simulink model "QP_lev2"  (R2022b)
settings: Solver=ode1  StartTime=0.0  StopTime=T_run  FixedStep=Ts  MaxStep=0.001  MinStep=0.001  RelTol=1e-3
InitFcn:
  | IMPC_Controller_simulink_initial
StopFcn:
  | Analyze
values from neighbouring files (symbols this model uses):
  A = [    A1       A2 ... (first row only)    [IMPC_Controller_simulink_initial.m]
  A_QP = reshape([W1;W2;W3;W4;I_bar]',m*n,1)    [IMPC_Controller_simulink_initial.m]
  B = [        B1 ... (first row only)    [IMPC_Controller_simulink_initial.m]
  D_bar_inv = inv(D_bar)    [IMPC_Controller_simulink_initial.m]
  d_gl = 1.0000    (= 1)    [IMPC_Controller_simulink_initial.m]
  d_l = 1.0000    (= 1)    [IMPC_Controller_simulink_initial.m]
  d_m_plus_d_g = 2.2036    [IMPC_Controller_simulink_initial.m]
  H_QP = reshape(H,((Nc))^2,1)    [IMPC_Controller_simulink_initial.m]
  K_b = Kb_coe*362    (= 362)    [IMPC_Controller_simulink_initial.m]
  L1_tilde = L1_bar*A_tilde    [IMPC_Controller_simulink_initial.m]
  L2_tilde = L2_bar*A_tilde    [IMPC_Controller_simulink_initial.m]
  L3_tilde = L3_bar*A_tilde    [IMPC_Controller_simulink_initial.m]
  L4_tilde = L4_bar*A_tilde    [IMPC_Controller_simulink_initial.m]
  lb_QP = dtau_min_bar    [IMPC_Controller_simulink_initial.m]
  lbA_QP_ini = [ repmat(q_min,N+1,1) ... (first row only)    [IMPC_Controller_simulink_initial.m]
  M_bar_inv = inv(M_bar)    [IMPC_Controller_simulink_initial.m]
  N = 10    [IMPC_Controller_simulink_initial.m]
  Q_const_pos_error = 8000    [IMPC_Controller_simulink_initial.m]
  Q_const_theta_error = 0    [IMPC_Controller_simulink_initial.m]
  Q_const_vel_error = 50    [IMPC_Controller_simulink_initial.m]
  q_sim_ini = q_ini    [IMPC_Controller_simulink_initial.m]
  R_const = 0.01    [IMPC_Controller_simulink_initial.m]
  tau_sim_ini = 0    [IMPC_Controller_simulink_initial.m]
  Ts = 0.001    [IMPC_Controller_simulink_initial.m]
  ub_QP = dtau_max_bar    [IMPC_Controller_simulink_initial.m]
  ubA_QP_ini = [ repmat(q_max,N+1,1) ... (first row only)    [IMPC_Controller_simulink_initial.m]
  var_u = 0    [IMPC_Controller_simulink_initial.m]
  var_y = 1e-12    [IMPC_Controller_simulink_initial.m]
  X_bar_sim_ini = [q_bar_sim_ini;theta_sim_ini;theta_d_sim_ini]    [IMPC_Controller_simulink_initial.m]
undefined symbols (not defined in the file or in its folder): C, D, exJoint, Xr
libraries: simulink x9, cstblocks x4
settings Model: PauseTimes=7.5  Creator=ywang  LastModifiedBy=zheng
settings SolverCC: InitialStep=0.001  AlgebraicLoopSolver=LineSearch
settings DataIOCC: ReturnWorkspaceOutputs=off
settings DebuggingCC: UnconnectedInputMsg=warning  UnconnectedOutputMsg=warning  UnconnectedLineMsg=warning  PregeneratedLibrarySubsystemCodeDiagnostic=none  SFMachineParentedDataDiag=warning  ArithmeticOperatorsInVariantConditions=warning
settings ModelReferenceCC: EnableRefExpFcnMdlSchedulingChecks=on
settings SFSimCC: SimUseLocalCustomCode=off  CustomCodeUndefinedFunction=UseInterfaceOnly
settings RTWCC: RTWUseLocalCustomCode=off  DLArmComputeVersion=19.05
settings CodeAppCC: StateflowObjectComments=on

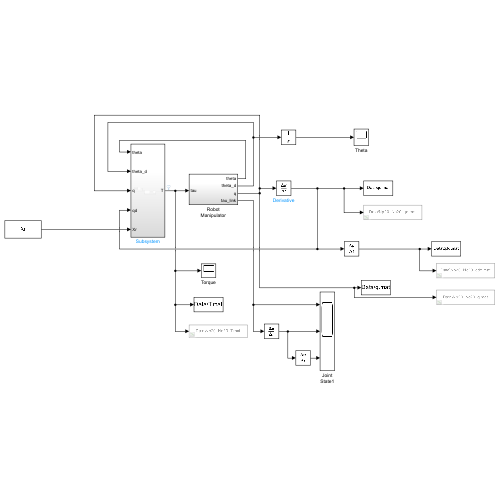
[thumbnail: Simulink's stored preview of the top-level diagram]
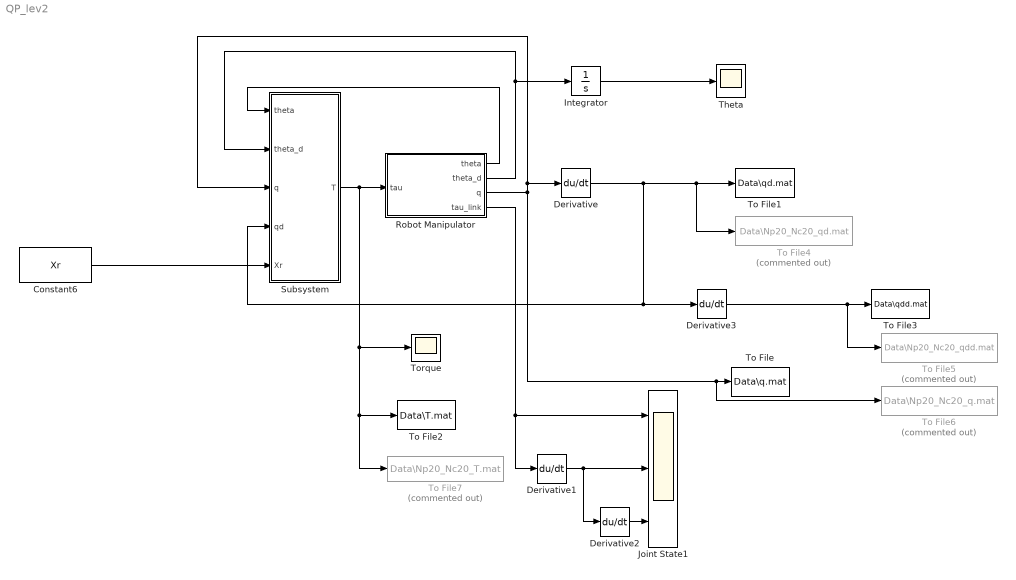
== system QP_lev2 ==
  Constant6 : Constant  Value=Xr
  Derivative{,1..3} (4 alike) : Derivative
  Integrator : Integrator
  Joint State1 : Scope  NumInputPorts=3
  Robot Manipulator : Subsystem
  Subsystem : Subsystem
  Theta : Scope
  To File : ToFile  Filename=Data\q.mat  MatrixName=q
  To File1 : ToFile  Filename=Data\qd.mat  MatrixName=qd
  To File2 : ToFile  Filename=Data\T.mat  MatrixName=T
  To File3 : ToFile  Filename=Data\qdd.mat  MatrixName=qdd
  To File4 : ToFile  Commented=on  Filename=Data\Np20_Nc20_qd.mat  MatrixName=Np20_Nc20_qd
  To File5 : ToFile  Commented=on  Filename=Data\Np20_Nc20_qdd.mat  MatrixName=Np20_Nc20_qdd
  To File6 : ToFile  Commented=on  Filename=Data\Np20_Nc20_q.mat  MatrixName=Np20_Nc20_q
  To File7 : ToFile  Commented=on  Filename=Data\Np20_Nc20_T.mat  MatrixName=Np20_Nc20_T
  Torque : Scope
  wires:
  Subsystem/1(T) -> To File7/1, To File2/1, Torque/1, Robot Manipulator/1(tau)
  Derivative/1 -> Derivative3/1, Subsystem/4(qd), To File4/1, To File1/1
  Robot Manipulator/3(q) -> Subsystem/3(q), Derivative/1, To File/1, To File6/1
  Constant6/1 -> Subsystem/5(Xr)
  Robot Manipulator/2(theta_d) -> Subsystem/2(theta_d), Integrator/1
  Integrator/1 -> Theta/1
  Robot Manipulator/4(tau_link) -> Derivative1/1, Joint State1/1
  Derivative1/1 -> Joint State1/2, Derivative2/1
  Derivative2/1 -> Joint State1/3
  Derivative3/1 -> To File5/1, To File3/1
  Robot Manipulator/1(theta) -> Subsystem/1(theta)

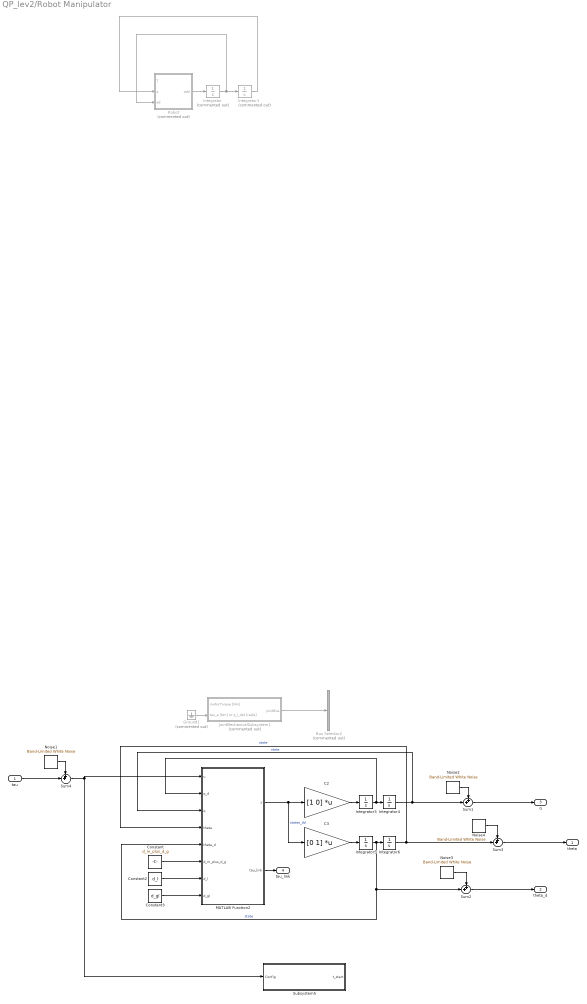
== system QP_lev2/Robot Manipulator ==
  tau : Inport  PortDimensions=1
  Bus Selector2 : BusSelector  Commented=on  OutputSignals=LinkPos,MotorPos,Torque
  C2 : Gain  Gain=[1 0]  Multiplication=Matrix(K*u)
  C3 : Gain  Gain=[0 1]  Multiplication=Matrix(K*u)
  Constant : Constant  Value=d_m_plus_d_g
  Constant2 : Constant  Value=d_l
  Constant3 : Constant  Value=d_gl
  Ground1 : Ground  Commented=on
  Integrator : Integrator  Commented=on  InitialCondition=[0;0;0]  ContinuousStateAttributes='velocity'
  Integrator1 : Integrator  Commented=on  InitialCondition=q_sim_ini  ContinuousStateAttributes='position'
  Integrator{3..6} (4 alike) : Integrator
  JointMechanicalSubsystem1 : Subsystem  Commented=on  AncestorBlock=cjt_library_models/Joint models/JointMechanicalSubsystem  mask(jointMechanicalSubsystem){jointObj=exJoint, fc_vel=1000, fc_torque=1000, input_delay=0, output_delay=1, quantize=off, quantize_bits=19, input_noise_enabled=off, output_noise_enabled=off, var_u=0, var_y=1.8e-10}
      mask prompts: jointObj "Joint Object"; fc_vel "Velocity filter cut-off frequency [Hz]"; fc_torque "Torque filter cut-off frequency [Hz]"; input_delay "Motor torque input delay (num samples of Ts)"; output_delay "Output delay (num samples of Ts)"; quantize "Quantize measurements"; quantize_bits "Quantization bits"; input_noise_enabled "Enable input noise"; output_noise_enabled "Enable measurement noise"; var_u "Input noise variance"; var_y "Measurement noise variance"
      mask help:
      | This block implements the mechanical dynamics of the actuator.
      |
      | For more information, see the > Help <.
      mask init:
      | % Get linear dynamics matrices
      | [A, B, C, D, I, R, K] = jointObj.getDynamicsMatrices();
      | 
      | % Build B matrix for nonlinear components
      | B_nonlinear = [zeros([size(B,1)-size(I,1),1]); 1./diag(I)];
      | 
      | % Get other properties
      | Ts      = jointObj.Ts;
      | Ts_elec = jointObj.Ts_elec;
      | k_b     = jointObj.k_b;
      | k_t     = jointObj.k_t;
      | n       = jointObj.n;
      | d_gl    = jointObj.d_gl;
      | 
      | % Handle MATLAB function block
      | handleMatlabFunctionBlock(gcb, jointObj);
      | 
      | % If input delay is enabled, set the flag to 1
      | input_delay_enable = 0;
      | if (input_delay > 0)
      |     input_delay_enable = 1;
      | end
      | 
      | % If noise is disabled, overwrite the given variances
      | if (input_noise_enabled == 0)
      |     var_u = 0;
      | end
      | if (output_noise_enabled == 0)
      | 	var_y = 0;
      | end
      settings: LibrarySourceBlock=cjt_library_models/Joint models/JointMechanicalSubsystem
      mask Help:
      | This block implements the mechanical dynamics of the actuator. Depending on the configuration in which the joint class was built, its dynamics are given by one of the variants provided by the toolbox (see model/linear/). If provided, the linear dynamics are enhanced with nonlinear components.
      | 
      | <b>Inputs</b>
      | <b>motorTorque</b>: Electromechanical motor torque provided on the rotor. An input delay can be added to this input (e.g. due to communication delays or a very simplified representation of electrical dynamics).
      | <b>tau_e or q_l_dot</b>: External interaction torque. Depending on the selected linear dynamics model of the joint, this is either the external torque acting on the load or the imposed load velocity (for fixed-output models).
      | 
      | <b>Outputs</b>
      | <b>jointBus</b>: The various variables and their measurements, with optional delays/noise/quantisation etc. For most outputs, several instances exist. Output variables ending in "NoNoise" denote physical quantities, without noise, filtering, or delays. All other variables are affected by noise and delays (if enabled). Lastly, variables ending in "Filtered" are also low-pass filtered, with cut-off frequency set in the mask.
      | 
      | <b>An important note with regards to output variables associated with torque.</b>
      | The "Torque" and "TorqueFiltered" are computed in the way torque is usually sensed by the control system; deflection times spring constant, i.e. only the stiffness contribution is considered, as usually the internal damping of the used flexible element (parameter d_gl) is very small. Hence, TorqueFiltered is used by the toolbox controllers as well.
      | However, as noted before, "TorqueNoNoise" denotes the physical quantity. This means that it includes the torque produced by internal damping of the elastic element (parameter d_gl).
      mask Callback quantize: toggleMaskFields(gcbh, 'quantize', 'quantize_bits');
      mask Callback input_noise_enabled: toggleMaskFields(gcbh, 'input_noise_enabled', 'var_u');
      mask Callback output_noise_enabled: toggleMaskFields(gcbh, 'output_noise_enabled', 'var_y');
  MATLAB Function2 : MATLAB Function  TreatAsAtomicUnit=on
  Noise1 : simulink/Sources/Band-Limited White Noise  Cov=var_u * Ts  Ts=Ts  seed=[3846513]
  Noise2 : simulink/Sources/Band-Limited White Noise  Cov=var_y * Ts  Ts=Ts  seed=[3846513]
  Noise3 : simulink/Sources/Band-Limited White Noise  Cov=var_y * Ts  Ts=Ts  seed=[3846513]
  Noise4 : simulink/Sources/Band-Limited White Noise  Cov=var_y * Ts  Ts=Ts  seed=[3846513]
  Robot : MATLAB Function  Commented=on  TreatAsAtomicUnit=on
  Subsystem5 : Subsystem
  Sum{1..4} (4 alike) : Sum  Inputs=++|
  theta : Outport
  theta_d : Outport  Port=2
  q : Outport  Port=3  VectorParamsAs1DForOutWhenUnconnected=off
  tau_link : Outport  Port=4
  wires:
  Integrator/1 -> Integrator1/1, Robot/3(qd)
  Integrator1/1 -> Robot/2(q)
  Robot/1(qdd) -> Integrator/1
  Ground1/1 -> JointMechanicalSubsystem1/2(tau_e [Nm] or q_l_dot [rad/s])
  JointMechanicalSubsystem1/1(jointBus) -> Bus Selector2/1
  MATLAB Function2/1(y) -> C3/1, C2/1  "states_dd"
  C3/1 -> Integrator5/1
  C2/1 -> Integrator3/1
  Integrator4/1 -> Sum1/2, MATLAB Function2/3(q)  "state"
  Integrator3/1 -> MATLAB Function2/2(q_d), Integrator4/1
  MATLAB Function2/2(tau_link) -> tau_link/1
  Sum4/1 -> MATLAB Function2/1(u), Subsystem5/1(Config)
  Noise1/1 -> Sum4/1
  tau/1 -> Sum4/2
  Noise2/1 -> Sum1/1
  Sum1/1 -> q/1
  Noise3/1 -> Sum2/1
  Integrator5/1 -> Sum2/2, MATLAB Function2/5(theta_d), Integrator6/1  "state"
  Sum2/1 -> theta_d/1
  Constant/1 -> MATLAB Function2/6(d_m_plus_d_g)
  Constant3/1 -> MATLAB Function2/8(d_gl)
  Constant2/1 -> MATLAB Function2/7(d_l)
  Sum3/1 -> theta/1
  Integrator6/1 -> Sum3/2, MATLAB Function2/4(theta)  "state"
  Noise4/1 -> Sum3/1

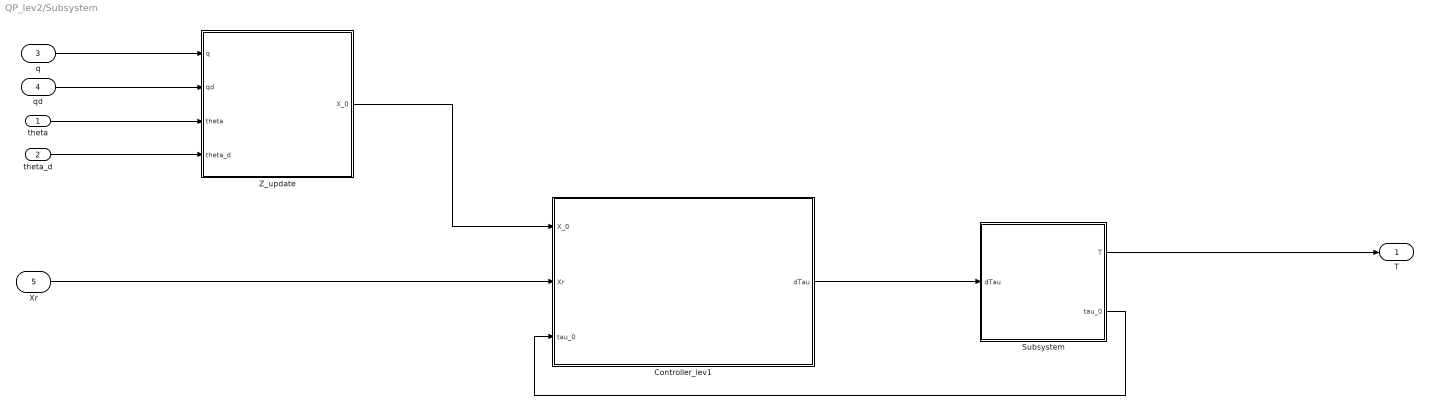
== system QP_lev2/Subsystem ==
  theta : Inport
  theta_d : Inport  Port=2
  q : Inport  Port=3
  qd : Inport  Port=4
  Xr : Inport  Port=5
  Controller_lev1 : Subsystem
  Subsystem : Subsystem
  Z_update : Subsystem
  T : Outport
  wires:
  q/1 -> Z_update/1(q)
  qd/1 -> Z_update/2(qd)
  Xr/1 -> Controller_lev1/2(Xr)
  Subsystem/1(T) -> T/1
  Subsystem/2(tau_0) -> Controller_lev1/3(tau_0)
  Z_update/1(X_0) -> Controller_lev1/1(X_0)
  Controller_lev1/1(dTau) -> Subsystem/1(dTau)
  theta_d/1 -> Z_update/4(theta_d)
  theta/1 -> Z_update/3(theta)

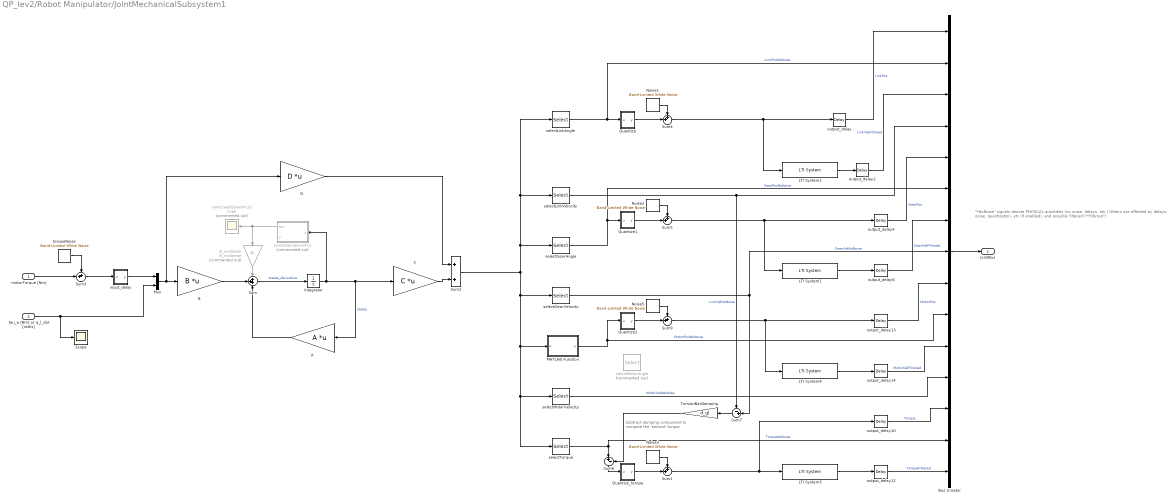
== system QP_lev2/Robot Manipulator/JointMechanicalSubsystem1 ==
  note: "*NoNoise" signals denote PHYSICAL quantities (no noise, delays, etc.)
      | Others are affected by delays, noise, quantization, etc (if enabled), and possibly filtered ("*Filtered")
  note: Subtract damping component to
      | compute the 'sensed' torque
  motorTorque [Nm] : Inport
  tau_e [Nm] or q_l_dot [rad/s] : Inport  Port=2
  A : Gain  Gain=A  Multiplication=Matrix(K*u)
  B : Gain  Gain=B  Multiplication=Matrix(K*u)
  B_nonlinear : Gain  Commented=on  Gain=B_nonlinear
  Bus Creator : BusCreator  Inputs=15
  C : Gain  Gain=C  Multiplication=Matrix(K*u)
  D : Gain  Gain=D  Multiplication=Matrix(K*u)
  Integrator : Integrator
  LTI System1 : cstblocks/LTI System  sys=c2d(tf([2*pi*fc_vel 0], [1 2*pi*fc_vel]), Ts, 'tustin')  IC=[]
  LTI System2 : cstblocks/LTI System  sys=c2d(tf([2*pi*fc_vel 0], [1 2*pi*fc_vel]), Ts, 'tustin')  IC=[]
  LTI System3 : cstblocks/LTI System  sys=c2d(tf([2*pi*fc_torque], [1 2*pi*fc_torque]), Ts, 'tustin')  IC=[]
  LTI System4 : cstblocks/LTI System  sys=c2d(tf([2*pi*fc_vel 0], [1 2*pi*fc_vel]), Ts, 'tustin')  IC=[]
  MATLAB Function : MATLAB Function  TreatAsAtomicUnit=on
  Mux : Mux  Inputs=2
  Noise1 : simulink/Sources/Band-Limited White Noise  Cov=var_y * Ts  Ts=Ts  seed=[3846513]
  Noise2 : simulink/Sources/Band-Limited White Noise  Cov=var_y * Ts  Ts=Ts  seed=[11563454]
  Noise3 : simulink/Sources/Band-Limited White Noise  Cov=jointObj.k_b^2 * sqrt(2) * var_y * Ts % sqrt(2) accounts for subtracting two encoders  Ts=Ts  seed=[960834]
  Noise5 : simulink/Sources/Band-Limited White Noise  Cov=var_y * Ts  Ts=Ts  seed=[24326]
  Quantize : Subsystem
  Quantize1 : Subsystem
  Quantize2 : Subsystem
  Quantize_torque : Subsystem
  Scope : Scope
  Sum : Sum  Inputs=+++
  Sum{1,3..5,9} (5 alike) : Sum  Inputs=++|
  Sum2 : Sum
  Sum6 : Sum  Inputs=|+-
  Sum7 : Sum  Inputs=-+|
  TorsionBarDamping : Gain  Gain=d_gl
  input_delay : Subsystem
  nonLinDynamicsFcn : MATLAB Function  Commented=on  TreatAsAtomicUnit=on
  nonLinearDynamicsScope : Scope  Commented=on
  output_delay{,2,4,6,10,12..14} (8 alike) : TransportDelay  DelayTime=output_delay * jointObj.Ts
  selectGearAngle : Selector  NumberOfDimensions=2  InputPortWidth=3  IndexOptions=Index vector (dialog),Select all  Indices=2,1  OutputSizes=1,1
  selectGearVelocity : Selector  NumberOfDimensions=2  InputPortWidth=3  IndexOptions=Index vector (dialog),Select all  Indices=5,1  OutputSizes=1,1
  selectLinkAngle : Selector  NumberOfDimensions=2  InputPortWidth=3  IndexOptions=Index vector (dialog),Select all  Indices=3,1  OutputSizes=1,1
  selectLinkVelocity : Selector  NumberOfDimensions=2  InputPortWidth=3  IndexOptions=Index vector (dialog),Select all  Indices=6,1  OutputSizes=1,1
  selectMotorAngle : Selector  Commented=on  NumberOfDimensions=2  InputPortWidth=3  IndexOptions=Index vector (dialog),Select all  Indices=1,1  OutputSizes=1,1
  selectMotorVelocity : Selector  NumberOfDimensions=2  InputPortWidth=3  IndexOptions=Index vector (dialog),Select all  Indices=4,1  OutputSizes=1,1
  selectTorque : Selector  NumberOfDimensions=2  InputPortWidth=3  IndexOptions=Index vector (dialog),Select all  Indices=7,1  OutputSizes=1,1
  torqueNoise : simulink/Sources/Band-Limited White Noise  Cov=var_u * Ts  Ts=Ts  seed=[2435345645]
  jointBus : Outport
  wires:
  Sum6/1 -> Quantize_torque/1(u)
  Noise3/1 -> Sum1/1
  Quantize_torque/1(y) -> Sum1/2
  Sum7/1 -> TorsionBarDamping/1
  TorsionBarDamping/1 -> Sum6/2
  C/1 -> Sum2/2
  D/1 -> Sum2/1
  Quantize2/1(y) -> Sum9/2
  Quantize1/1(y) -> Sum5/2
  Quantize/1(y) -> Sum4/2
  Sum1/1 -> LTI System3/1, output_delay10/1
  LTI System3/1 -> output_delay12/1
  tau_e [Nm] or q_l_dot [rad/s]/1 -> Scope/1, Mux/2
  Mux/1 -> B/1, D/1
  Sum9/1 -> output_delay13/1, LTI System4/1
  output_delay14/1 -> Bus Creator/11  "MotorVelFiltered"
  output_delay13/1 -> Bus Creator/9  "MotorPos"
  LTI System4/1 -> output_delay14/1
  Noise5/1 -> Sum9/1
  output_delay12/1 -> Bus Creator/15  "TorqueFiltered"
  selectTorque/1 -> Bus Creator/14, Sum6/1  "TorqueNoNoise"
  output_delay10/1 -> Bus Creator/13  "Torque"
  selectMotorVelocity/1 -> Bus Creator/12  "MotorVelNoNoise"
  MATLAB Function/1(y) -> Bus Creator/10, Quantize2/1(u)  "MotorPosNoNoise"
  selectGearVelocity/1 -> Sum7/2, Bus Creator/8  "GearVelNoNoise"
  output_delay6/1 -> Bus Creator/7  "GearVelFiltered"
  selectGearAngle/1 -> Quantize1/1(u), Bus Creator/6  "GearPosNoNoise"
  output_delay4/1 -> Bus Creator/5  "GearPos"
  selectLinkVelocity/1 -> Sum7/1, Bus Creator/4  "LinkVelNoNoise"
  output_delay2/1 -> Bus Creator/3  "LinkVelFiltered"
  selectLinkAngle/1 -> Bus Creator/2, Quantize/1(u)  "LinkPosNoNoise"
  output_delay/1 -> Bus Creator/1  "LinkPos"
  A/1 -> Sum/3
  B/1 -> Sum/2
  Integrator/1 -> A/1, C/1, nonLinDynamicsFcn/1(x)  "states"
  motorTorque [Nm]/1 -> Sum3/2
  LTI System2/1 -> output_delay2/1
  Sum/1 -> Integrator/1  "states_derivative"
  LTI System1/1 -> output_delay6/1
  Noise1/1 -> Sum4/1
  Noise2/1 -> Sum5/1
  torqueNoise/1 -> Sum3/1
  Sum4/1 -> output_delay/1, LTI System2/1
  Sum5/1 -> output_delay4/1, LTI System1/1
  Sum3/1 -> input_delay/1(u)
  input_delay/1(y) -> Mux/1
  Bus Creator/1 -> jointBus/1
  nonLinDynamicsFcn/1(tau) -> B_nonlinear/1, nonLinearDynamicsScope/1
  B_nonlinear/1 -> Sum/1
  Sum2/1 -> MATLAB Function/1(u), selectMotorVelocity/1, selectTorque/1, selectGearVelocity/1, selectGearAngle/1, selectLinkVelocity/1, selectLinkAngle/1

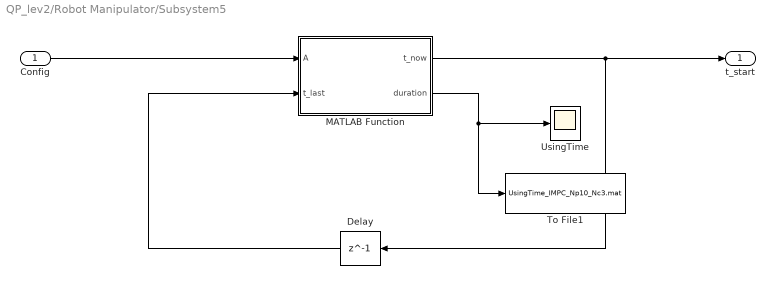
== system QP_lev2/Robot Manipulator/Subsystem5 ==
  Config : Inport
  Delay : Delay  DelayLength=1  InitialCondition=[0 0]
  MATLAB Function : MATLAB Function  TreatAsAtomicUnit=on
  To File1 : ToFile  Filename=UsingTime_IMPC_Np10_Nc3.mat  MatrixName=UsingTime_IMPC_Np10_Nc3
  UsingTime : Scope
  t_start : Outport
  wires:
  MATLAB Function/1(t_now) -> Delay/1, t_start/1
  Config/1 -> MATLAB Function/1(A)
  Delay/1 -> MATLAB Function/2(t_last)
  MATLAB Function/2(duration) -> To File1/1, UsingTime/1

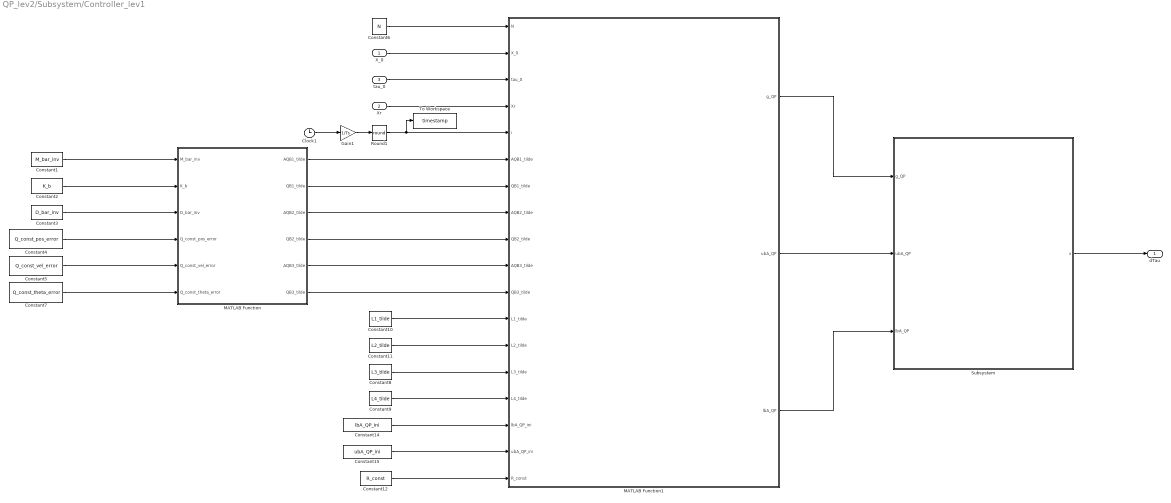
== system QP_lev2/Subsystem/Controller_lev1 ==
  X_0 : Inport
  Xr : Inport  Port=2
  tau_0 : Inport  Port=3
  Clock1 : Clock
  Constant1 : Constant  Value=M_bar_inv
  Constant10 : Constant  Value=L1_tilde
  Constant11 : Constant  Value=L2_tilde
  Constant12 : Constant  Value=R_const
  Constant14 : Constant  Value=lbA_QP_ini
  Constant15 : Constant  Value=ubA_QP_ini
  Constant2 : Constant  Value=K_b
  Constant3 : Constant  Value=D_bar_inv
  Constant4 : Constant  Value=Q_const_pos_error
  Constant5 : Constant  Value=Q_const_vel_error
  Constant6 : Constant  Value=N
  Constant7 : Constant  Value=Q_const_theta_error
  Constant8 : Constant  Value=L3_tilde
  Constant9 : Constant  Value=L4_tilde
  Gain1 : Gain  Gain=1/Ts
  MATLAB Function : MATLAB Function  TreatAsAtomicUnit=on
  MATLAB Function1 : MATLAB Function  TreatAsAtomicUnit=on
  Round1 : Rounding  Operator=round
  Subsystem : Subsystem
  To Workspace : ToWorkspace  VariableName=timestamp  SaveFormat=Timeseries  SampleTime=-1
  dTau : Outport
  wires:
  Constant11/1 -> MATLAB Function1/13(L2_tilde)
  Constant10/1 -> MATLAB Function1/12(L1_tilde)
  MATLAB Function1/1(g_QP) -> Subsystem/1(g_QP)
  Round1/1 -> MATLAB Function1/5(i), To Workspace/1
  Clock1/1 -> Gain1/1
  Gain1/1 -> Round1/1
  Xr/1 -> MATLAB Function1/4(Xr)
  Constant14/1 -> MATLAB Function1/16(lbA_QP_ini)
  Constant15/1 -> MATLAB Function1/17(ubA_QP_ini)
  Constant6/1 -> MATLAB Function1/1(N)
  Subsystem/1(x) -> dTau/1
  MATLAB Function1/3(lbA_QP) -> Subsystem/3(lbA_QP)
  MATLAB Function1/2(ubA_QP) -> Subsystem/2(ubA_QP)
  X_0/1 -> MATLAB Function1/2(X_0)
  tau_0/1 -> MATLAB Function1/3(tau_0)
  Constant12/1 -> MATLAB Function1/18(R_const)
  Constant7/1 -> MATLAB Function/6(Q_const_theta_error)
  Constant5/1 -> MATLAB Function/5(Q_const_vel_error)
  Constant4/1 -> MATLAB Function/4(Q_const_pos_error)
  Constant3/1 -> MATLAB Function/3(D_bar_inv)
  Constant2/1 -> MATLAB Function/2(K_b)
  Constant1/1 -> MATLAB Function/1(M_bar_inv)
  MATLAB Function/1(AQB1_tilde) -> MATLAB Function1/6(AQB1_tilde)
  MATLAB Function/2(QB1_tilde) -> MATLAB Function1/7(QB1_tilde)
  MATLAB Function/3(AQB2_tilde) -> MATLAB Function1/8(AQB2_tilde)
  MATLAB Function/4(QB2_tilde) -> MATLAB Function1/9(QB2_tilde)
  MATLAB Function/5(AQB3_tilde) -> MATLAB Function1/10(AQB3_tilde)
  MATLAB Function/6(QB3_tilde) -> MATLAB Function1/11(QB3_tilde)
  Constant8/1 -> MATLAB Function1/14(L3_tilde)
  Constant9/1 -> MATLAB Function1/15(L4_tilde)

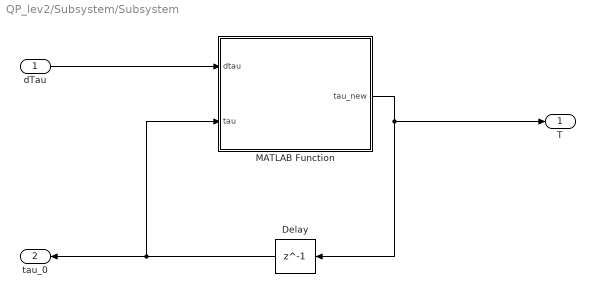
== system QP_lev2/Subsystem/Subsystem ==
  dTau : Inport
  Delay : Delay  DelayLength=1  InitialCondition=tau_sim_ini
  MATLAB Function : MATLAB Function  TreatAsAtomicUnit=on
  T : Outport
  tau_0 : Outport  Port=2
  wires:
  dTau/1 -> MATLAB Function/1(dtau)
  Delay/1 -> MATLAB Function/2(tau), tau_0/1
  MATLAB Function/1(tau_new) -> T/1, Delay/1

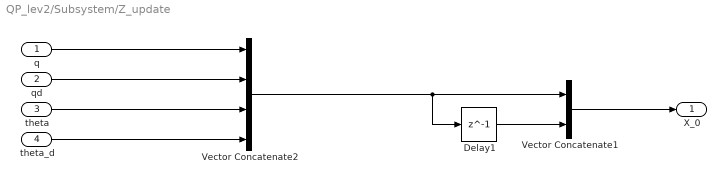
== system QP_lev2/Subsystem/Z_update ==
  q : Inport
  qd : Inport  Port=2
  theta : Inport  Port=3
  theta_d : Inport  Port=4
  Delay1 : Delay  DelayLength=1  InitialCondition=X_bar_sim_ini
  Vector Concatenate1 : Concatenate
  Vector Concatenate2 : Concatenate  NumInputs=4
  X_0 : Outport
  wires:
  qd/1 -> Vector Concatenate2/2
  q/1 -> Vector Concatenate2/1
  Vector Concatenate1/1 -> X_0/1
  Delay1/1 -> Vector Concatenate1/2
  Vector Concatenate2/1 -> Delay1/1, Vector Concatenate1/1
  theta_d/1 -> Vector Concatenate2/4
  theta/1 -> Vector Concatenate2/3

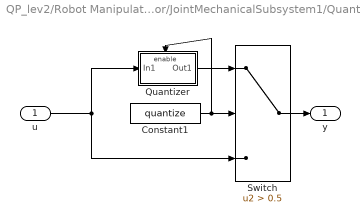
== system QP_lev2/Robot Manipulator/JointMechanicalSubsystem1/Quantize ==
  u : Inport
  Constant1 : Constant  Value=quantize
  Quantizer : Subsystem
  Switch : Switch  Criteria=u2 > Threshold  Threshold=0.5  SaturateOnIntegerOverflow=off  InputSameDT=off
  y : Outport
  wires:
  u/1 -> Quantizer/1(In1), Switch/3
  Constant1/1 -> Quantizer/Enable, Switch/2
  Switch/1 -> y/1
  Quantizer/1(Out1) -> Switch/1

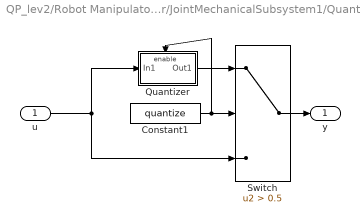
== system QP_lev2/Robot Manipulator/JointMechanicalSubsystem1/Quantize1 ==
  u : Inport
  Constant1 : Constant  Value=quantize
  Quantizer : Subsystem
  Switch : Switch  Criteria=u2 > Threshold  Threshold=0.5  SaturateOnIntegerOverflow=off  InputSameDT=off
  y : Outport
  wires:
  u/1 -> Quantizer/1(In1), Switch/3
  Constant1/1 -> Quantizer/Enable, Switch/2
  Switch/1 -> y/1
  Quantizer/1(Out1) -> Switch/1

== system QP_lev2/Robot Manipulator/JointMechanicalSubsystem1/Quantize2 ==
  u : Inport
  Constant1 : Constant  Value=quantize
  Quantizer : Subsystem
  Switch : Switch  Criteria=u2 > Threshold  Threshold=0.5  SaturateOnIntegerOverflow=off  InputSameDT=off
  y : Outport
  wires:
  u/1 -> Quantizer/1(In1), Switch/3
  Constant1/1 -> Quantizer/Enable, Switch/2
  Switch/1 -> y/1
  Quantizer/1(Out1) -> Switch/1

== system QP_lev2/Robot Manipulator/JointMechanicalSubsystem1/Quantize_torque ==
  note: This quantizer uses the stiffness to scale the quantisation.
      | This signal should *not* be used for nonlinear stiffness!
  u : Inport
  Constant1 : Constant  Value=quantize
  Quantizer : Subsystem
  Switch : Switch  Criteria=u2 > Threshold  Threshold=0.5  SaturateOnIntegerOverflow=off  InputSameDT=off
  y : Outport
  wires:
  Quantizer/1(Out1) -> Switch/1
  Switch/1 -> y/1
  Constant1/1 -> Switch/2, Quantizer/Enable
  u/1 -> Switch/3, Quantizer/1(In1)

== system QP_lev2/Robot Manipulator/JointMechanicalSubsystem1/input_delay ==
  u : Inport
  Constant1 : Constant  Value=input_delay_enable
  Switch : Switch  Criteria=u2 > Threshold  SaturateOnIntegerOverflow=off  InputSameDT=off
  delay : Subsystem
  y : Outport
  wires:
  u/1 -> delay/1(In1), Switch/3
  Constant1/1 -> Switch/2, delay/Enable
  Switch/1 -> y/1
  delay/1(Out1) -> Switch/1

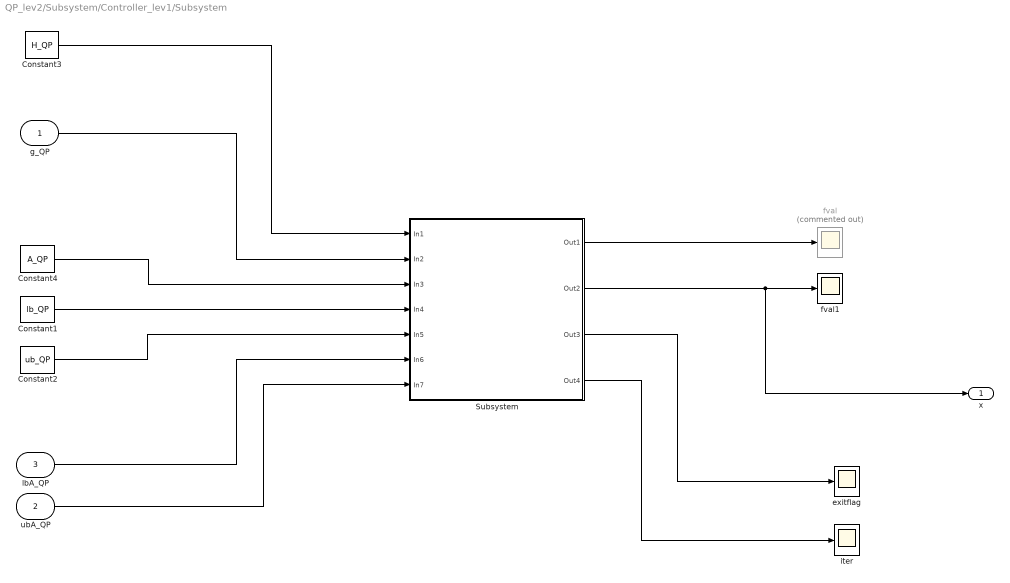
== system QP_lev2/Subsystem/Controller_lev1/Subsystem ==
  g_QP : Inport  PortDimensions=3
  ubA_QP : Inport  Port=2  PortDimensions=47
  lbA_QP : Inport  Port=3  PortDimensions=47
  Constant1 : Constant  Value=lb_QP
  Constant2 : Constant  Value=ub_QP
  Constant3 : Constant  Value=H_QP
  Constant4 : Constant  Value=A_QP
  Subsystem : Subsystem
  exitflag : Scope
  fval : Scope  Commented=on
  fval1 : Scope
  iter : Scope
  x : Outport
  wires:
  Subsystem/2(Out2) -> fval1/1, x/1
  Constant3/1 -> Subsystem/1(In1)
  g_QP/1 -> Subsystem/2(In2)
  Constant4/1 -> Subsystem/3(In3)
  lbA_QP/1 -> Subsystem/6(In6)
  ubA_QP/1 -> Subsystem/7(In7)
  Subsystem/1(Out1) -> fval/1
  Subsystem/3(Out3) -> exitflag/1
  Subsystem/4(Out4) -> iter/1
  Constant1/1 -> Subsystem/4(In4)
  Constant2/1 -> Subsystem/5(In5)

== system QP_lev2/Robot Manipulator/JointMechanicalSubsystem1/Quantize/Quantizer ==
  In1 : Inport
  Enable : EnablePort
  Quantizer : Quantizer  QuantizationInterval=1/(2^quantize_bits)
  Out1 : Outport
  wires:
  In1/1 -> Quantizer/1
  Quantizer/1 -> Out1/1

== system QP_lev2/Robot Manipulator/JointMechanicalSubsystem1/Quantize1/Quantizer ==
  In1 : Inport
  Enable : EnablePort
  Quantizer : Quantizer  QuantizationInterval=1/(2^quantize_bits)
  Out1 : Outport
  wires:
  In1/1 -> Quantizer/1
  Quantizer/1 -> Out1/1

== system QP_lev2/Robot Manipulator/JointMechanicalSubsystem1/Quantize2/Quantizer ==
  In1 : Inport
  Enable : EnablePort
  Quantizer : Quantizer  QuantizationInterval=1/(2^quantize_bits)
  Out1 : Outport
  wires:
  In1/1 -> Quantizer/1
  Quantizer/1 -> Out1/1

== system QP_lev2/Robot Manipulator/JointMechanicalSubsystem1/Quantize_torque/Quantizer ==
  In1 : Inport
  Enable : EnablePort
  Quantizer : Quantizer  QuantizationInterval=jointObj.k_b * (1/(2^quantize_bits))
  Out1 : Outport
  wires:
  Quantizer/1 -> Out1/1
  In1/1 -> Quantizer/1

== system QP_lev2/Robot Manipulator/JointMechanicalSubsystem1/input_delay/delay ==
  note: The delay value here is computed so that it is >0 when delay is DISABLED,
      | to avoid MATLAB throwing warnings unnecessarily.
  In1 : Inport
  Enable : EnablePort
  input_delay : TransportDelay  DelayTime=input_delay * jointObj.Ts + 1 - input_delay_enable  TransDelayFeedthrough=on
  Out1 : Outport
  wires:
  In1/1 -> input_delay/1
  input_delay/1 -> Out1/1

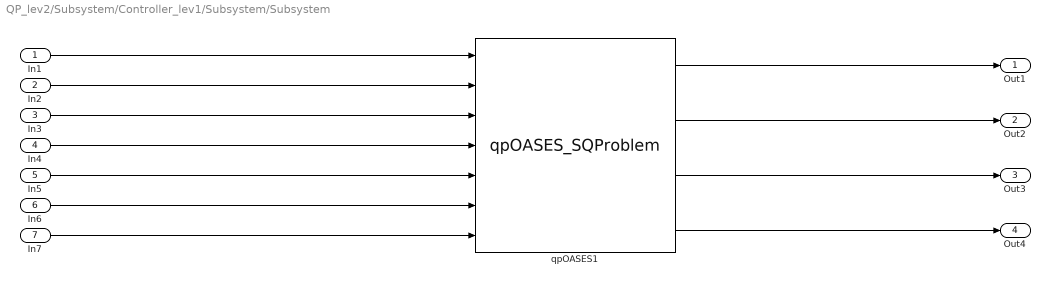
== system QP_lev2/Subsystem/Controller_lev1/Subsystem/Subsystem ==
  In1 : Inport
  In2 : Inport  Port=2
  In3 : Inport  Port=3
  In4 : Inport  Port=4
  In5 : Inport  Port=5
  In6 : Inport  Port=6
  In7 : Inport  Port=7
  qpOASES1 : S-Function  FunctionName=qpOASES_SQProblem  SFunctionDeploymentMode=off  EnableBusSupport=off
  Out1 : Outport
  Out2 : Outport  Port=2
  Out3 : Outport  Port=3
  Out4 : Outport  Port=4
  wires:
  qpOASES1/4 -> Out4/1
  In1/1 -> qpOASES1/1
  qpOASES1/3 -> Out3/1
  In2/1 -> qpOASES1/2
  In7/1 -> qpOASES1/7
  In4/1 -> qpOASES1/4
  In3/1 -> qpOASES1/3
  qpOASES1/2 -> Out2/1
  qpOASES1/1 -> Out1/1
  In6/1 -> qpOASES1/6
  In5/1 -> qpOASES1/5

== matlab function QP_lev2/Subsystem/Subsystem/MATLAB Function ==
  data: dtau input; tau_new output; tau input
function tau_new   = fcn(dtau,tau)
%     tau_new = tau+dtau(1:3);
    tau_new = tau+dtau(1);
%     tau_new_one = tau_new(1);
    
%     tau_new_first = tau(3)+dtau(3);
%     tau_new = [0;0;tau_new_first];

%     tau_new = dtau(1:3);

end

== matlab function QP_lev2/Robot Manipulator/Subsystem5/MATLAB Function ==
  data: A input; t_now output; t_last input; duration output
function [t_now, duration] = fcn(A, t_last)
    tStart = tic;
    t_now = [tStart.tv_sec, tStart.tv_nsec];
    
    duration = tStart.tv_sec-t_last(1) + (tStart.tv_nsec-t_last(2))*10^-9;
    
end

== matlab function QP_lev2/Subsystem/Controller_lev1/MATLAB Function ==
  data: M_bar_inv input; AQB1_tilde output; K_b input; D_bar_inv input; Q_const_pos_error input; Q_const_vel_error input; Q_const_theta_error input; QB1_tilde output; AQB2_tilde output; QB2_tilde output; AQB3_tilde output; QB3_tilde output
function [AQB1_tilde,QB1_tilde,AQB2_tilde,QB2_tilde,AQB3_tilde,QB3_tilde]= fcn(M_bar_inv,K_b,D_bar_inv,Q_const_pos_error,Q_const_vel_error,Q_const_theta_error)

N = 10;
Nc = 3;
Ts = 0.001; 

A1_a22 = 2-M_bar_inv*K_b*Ts*Ts;
A1 = [1    Ts       0        0;
      0   A1_a22    0   M_bar_inv*K_b*Ts*Ts;
      0    0        1        Ts;
      0    0        0        2];
A2 = [0    0    0    0;
      0   -1    0    0;
      0    0    0    0;
      0    0    0   -1];
B1 = [0;
      0;
      0;
      D_bar_inv*Ts];
  
A = [    A1       A2;
     eye(4) zeros(4)];
B = [        B1;
     zeros(4,1)];

A_tilde = Formulate_N_PowerMatVector(N, A);%8(N+1)x8
B_tilde = Formulate_N_RecurMat_Nc(N,Nc, A,B);%8(N+1)xNc



K1_bar = [1 0 0 0 0 0 0 0];%1x8
K2_bar = [0 1 0 0 0 0 0 0];%1x8
K3_bar = [0 0 0 1 0 0 0 0];%1x8


U1_bar = K1_bar'*Q_const_pos_error*K1_bar;%8x8
Q1_tilde = Formulate_N_BlkdiagMat(N+1, U1_bar);%8Nx8N
U2_bar = K2_bar'*Q_const_vel_error*K2_bar;%8x8
Q2_tilde = Formulate_N_BlkdiagMat(N+1, U2_bar);%8Nx8N
U3_bar = K3_bar'*Q_const_theta_error*K3_bar;%8x8
Q3_tilde = Formulate_N_BlkdiagMat(N+1, U3_bar);%8Nx8N


Ud1_bar = Q_const_pos_error*K1_bar;%1x8
AQB_tilde = zeros(8,Nc);
QB_tilde = zeros(N+1,Nc);
QB1_tilde = Formulate_N_BlkdiagMat(N+1, Ud1_bar)*B_tilde+QB_tilde;%(N+1)x8(N+1) * 8(N+1)xNc = (N+1)xNc
AQB1_tilde = A_tilde'*Q1_tilde*B_tilde+AQB_tilde;%8xNc

Ud2_bar = Q_const_vel_error*K2_bar;%1x8
AQB_tilde = zeros(8,Nc);
QB_tilde = zeros(N+1,Nc);
QB2_tilde = Formulate_N_BlkdiagMat(N+1, Ud2_bar)*B_tilde+QB_tilde;%(N+1)x8(N+1) * 8(N+1)xNc = (N+1)xNc
AQB2_tilde = A_tilde'*Q2_tilde*B_tilde+AQB_tilde;%8xNc

Ud3_bar = Q_const_theta_error*K3_bar;%1x8
AQB_tilde = zeros(8,Nc);
QB_tilde = zeros(N+1,Nc);
QB3_tilde = Formulate_N_BlkdiagMat(N+1, Ud3_bar)*B_tilde+QB_tilde;%(N+1)x8(N+1) * 8(N+1)xNc = (N+1)xNc
AQB3_tilde = A_tilde'*Q3_tilde*B_tilde+AQB_tilde;%8xNc



% AQB_tilde = zeros(6,N);
% QB_tilde = zeros(2*N,N);
% QB_tilde = Formulate_N_BlkdiagMat(N, Ud_bar)*B_tilde+QB_tilde;%2Nx6N * 6NxN = 2NxN
% AQB_tilde = A_tilde'*Q_tilde*B_tilde+AQB_tilde;%6xN

== matlab function QP_lev2/Subsystem/Controller_lev1/MATLAB Function1 ==
  settings: updateMethod=DISCRETE
  data: N input; X_0 input; tau_0 input; Xr input; i input; AQB1_tilde input; QB1_tilde input; AQB2_tilde input; QB2_tilde input; AQB3_tilde input; QB3_tilde input; L1_tilde input; L2_tilde input; L3_tilde input; L4_tilde input; g_QP output; ubA_QP output; lbA_QP output; lbA_QP_ini input; ubA_QP_ini input; R_const input
function [g_QP, ubA_QP, lbA_QP] = QP_parameter(N, X_0,tau_0, Xr,i, AQB1_tilde,QB1_tilde,AQB2_tilde,QB2_tilde,AQB3_tilde,QB3_tilde, L1_tilde,L2_tilde,L3_tilde,L4_tilde,lbA_QP_ini,ubA_QP_ini,R_const)
    k = 10;
    kc = 3;
    Ts = 0.001;

    tau_0_bar = repmat(tau_0,kc,1); 
%     Xr_0 = Xr(:,i+1:i+k);%2xN
    Xr_0_bar = reshape(Xr(1,i+1:i+k+1),N+1,1);
    Xr_0_bar_dot = reshape(Xr(2,i+1:i+k+1),N+1,1);
    Xr_0_theta_dot = reshape(Xr(3,i+1:i+k+1),N+1,1);

    

    g_QP_ = X_0'*AQB1_tilde-Xr_0_bar'*QB1_tilde+X_0'*AQB2_tilde-Xr_0_bar_dot'*QB2_tilde+X_0'*AQB3_tilde-Xr_0_theta_dot'*QB3_tilde;%1xNc
    g_QP = 2*g_QP_';

    
%     delta_tau_ref = delta_tau_ref_total(i+1:i+k);
%     delta_tau_ref_ = reshape(delta_tau_ref,1,k);
%     matrix_uref_qd = delta_tau_ref_*R_const;
%     g_QP = X_0'*AQB_tilde-Xr_0_bar'*QB_tilde-matrix_uref_qd;%1x10
    
    % with qd constraints
    bA_QP = [L1_tilde*X_0;
             L2_tilde*X_0;
             L3_tilde*X_0;
             L4_tilde*X_0;
                tau_0_bar];
    
    lbA_QP = lbA_QP_ini-bA_QP;
    ubA_QP = ubA_QP_ini-bA_QP;
    
    
end

== matlab function QP_lev2/Robot Manipulator/Robot ==
  data: T input; qdd output; q input; qd input
function qdd = fcn(T,q,qd)
%#codegen

% cos and sine
c2 = cos(q(2));
c3 = cos(q(3));
c23 = cos(q(2)+q(3));
s2 = sin(q(2));
s3 = sin(q(3));
s23 = sin(q(2)+q(3));
% M-components
m11 = 1.0425+0.08094*c23+0.3484*c2+.0561*c3;
m12 = 0.4398+.04047*c23+.1742*c2+.0561*c3;
m13 = .1788+.04047*c23+.02809*c3;
m22 = .4398+.0519*c3;
m23 = .1788+.02809*c3;
m33 = .1788;
% Mass-Inertia matrix
M = [m11 m12 m13;
     m12 m22 m23;
     m13 m23 m33];
% N-components
n11 = -.1742*s2*qd(2)^2-0.04047*s23*qd(2)^2-.02809*s3*qd(3)^2-.04047*s23*qd(3)^2-0.3484*s2*qd(1)*qd(2)-.08094*s23*qd(1)*qd(2);
n12 = -0.05619*s3*qd(1)*qd(3)-.08094*s23*qd(1)*qd(3)-.05619*s3*qd(2)*qd(3)-.08094*s23*qd(2)*qd(3);
n2 = .1742*s2*qd(1)^2+.04047*s23*qd(1)^2-.02809*s3*qd(3)^2-0.0561*s3*qd(1)*qd(3)-0.05619*s3*qd(2)*qd(3);
n3 = 0.02809*s3*qd(1)^2+.02809*s3*qd(2)^2+.04047*s23*qd(1)^2+.05619*s3*qd(1)*qd(2);
% N matrix
N = [n11+n12;
     n2;
     n3];
% Friction coefficients
F = [2.6e-4 0 0;
     0 2.6e-4 0; 
     0 0 2.6e-4];

qdd=M\(T-N-F*qd);

== matlab function QP_lev2/Robot Manipulator/JointMechanicalSubsystem1/nonLinDynamicsFcn ==
  data: tau output; x input; y output
function [tau, y] = nonLinDynamics(x)
%#codegen

params.a_CU = 0.003900;
params.c_CU = 380.000000;
params.c_FE = 460.000000;
params.diam = 93.000000;
params.len = 163.000000;
params.m = 1.000000;
params.I_m = 0.230000;
params.I_g = 0.368000;
params.I_l = 1.000000;
params.k_g = 31000.000000;
params.k_b = 362.000000;
params.d_m = 0.000000;
params.d_g = 0.000000;
params.d_l = 0.000000;
params.d_m_n = 14.786000;
params.d_g_n = 0.000000;
params.d_l_n = 0.000000;
params.d_mg = 300.000000;
params.d_gl = 0.000000;
params.d_cm = 0.000000;
params.d_cg = 0.000000;
params.d_cl = 0.000000;
params.d_cm_n = 0.185800;
params.d_cg_n = 0.000000;
params.d_cl_n = 0.000000;
params.d_s = 0.000000;
params.v_s = 0.000000;
params.rip_types = [];
params.rip_a1 = [];
params.rip_a2 = [];
params.rip_f = [];
params.n = 100.000000;
params.k_t = 0.078000;
params.r = 0.318000;
params.x = 0.000200;
params.p = 6.000000;
params.v_0 = 24.000000;
params.i_p = 80.000000;
params.dq_p = 5.860000;
params.r_th1 = 0.290000;
params.r_th2 = 3.450000;
params.T_thw = 3.960000;
params.T_thm = 1240.000000;
params.Tmp_WMax = 120.000000;
params.Tmp_ANom = 25.000000;
params.name = 'Example_Joint';
params.paramName = 'my_param';
params.modelName = 'rigid_gearbox';
params.nonlinearModelName = 'coulomb';
params.electricalModelName = 'electric_dyn';
params.Ts = 0.001000;
params.Ts_elec = 0.000100;
[tau, y] =coulomb(params,x);
	end

== matlab function QP_lev2/Robot Manipulator/JointMechanicalSubsystem1/MATLAB Function ==
  data: u input; y output
function y = fcn(u)

y = u(1);

== matlab function QP_lev2/Robot Manipulator/MATLAB Function2 ==
  data: u input; q_d input; q input; theta input; theta_d input; y output; tau_link output; d_m_plus_d_g input; d_l input; d_gl input
function [y,tau_link] = fcn(u,   q_d, q,theta,theta_d,d_m_plus_d_g,d_l,d_gl)
K_b = 362;
% K_b = 100;
% K_b = 6000;
M = 1;
D = 0.598;
% D = 1;
% g = 9.81;
% L = 1;
% m = 1;

% % Linear viscous friction
% d_m = 0.0036;  %% Motor Damping [Nms/rad]
% d_g = 2.2000;  %% Gearbox damping [Nms/rad]
% d_l = 0.0000;  %% Torsion bar damping [Nms/rad]

% % Linear internal viscous friction
% d_gl = 0.0000;  %% Torsion bar internal damping [Nms/rad] (not identified)



y = zeros(2,1);


% nonlinearPart = -(m*g*L)/M;

y(1) = (K_b/M)*(theta-q)+(d_gl/M)*(theta_d-q_d)-d_l*q_d;

y(2) =  (K_b/D)*(q-theta)+(d_gl/D)*(q_d-theta_d)-(d_m_plus_d_g)*theta_d+(u/D);


tau_link = K_b*(theta-q);
